simulink model "sm_DynamicCompression"  (R2019b)
settings: Solver=FixedStepDiscrete  StartTime=0.0  StopTime=stop_time  RelTol=1e-3
InitFcn:
  | sm_callback_init
StopFcn:
  | sm_callback_stop
values from neighbouring files (symbols this model uses):
  a = 100*(r^2)    [InitializeCompressionSettings.m]    (also in sm_check_control_signals.m = registers(i).(supplied_fields{j}); sm_check_control_signals_LOCAL_1434.m = registers(i).(supplied_fields{j}))
  B_k_0_init = zeros(1,FIR_0_Uprate)    [sm_callback_init.m]
  B_k_1_init = zeros(1,FIR_0_Uprate)    [sm_callback_init.m]
  B_k_2_init = zeros(1,FIR_0_Uprate)    [sm_callback_init.m]
  B_k_3_init = zeros(1,FIR_0_Uprate)    [sm_callback_init.m]
  B_k_4_init = zeros(1,FIR_0_Uprate)    [sm_callback_init.m]
  B_k_5_init = zeros(1,FIR_0_Uprate)    [sm_callback_init.m]
  calib_bpfs = bpfs    [sm_compression_init.m]
  delayFix = maxDelay-delays    [Initialize_Delay_Values.m]
  F_bits = 28    [TestingLibraryScripts.m]    (also in sm_compression_init.m)
  FIR_0_Size = (ceil(log2(length(calib_bpfs(2:calib_bpfs(1,1)+1 ,1)'))))    [sm_callback_init.m]
  FIR_0_Uprate = 2^FIR_0_Size    [sm_callback_init.m]
  M_bits = 1    [TestingLibraryScripts.m]    (also in sm_compression_init.m = 5)
  M_Bits = M_bits    (= 5)    [sm_compression_init.m]
  mp = sm_init_avalon_signals(mp)    [sm_callback_init.m]
  r_att = nthroot(0.1, s_att)    [sm_compression_init.m]
  r_rel = nthroot(0.1, s_rel)    [sm_compression_init.m]
  recombGain = ones(1,NChans)    [sm_compression_init.m]
  TABLE_SEL_BYPASS_ENABLE = 0    [sm_callback_init.m]
  Ts = mp.Ts    [sm_compression_init.m]
  Ts_system = mp.Ts_system    [sm_compression_init.m]
  W_bits = 32    [TestingLibraryScripts.m]    (also in sm_compression_init.m)
  X_high = 1    [sm_compression_init.m]
undefined symbols (not defined in the file or in its folder): b, c, Gain_Table, ig_eq
libraries: hdlsllib x272, simulink x127, dsphdlfiltering x2
(part 1 of 8)
settings Model: Creator=Ross  LastModifiedBy=cb54103
settings DataIOCC: ReturnWorkspaceOutputs=off
settings OptimizationCC: BlockReduction=off  ConditionallyExecuteInputs=off  DefaultParameterBehavior=Inlined
settings DebuggingCC: ReadBeforeWriteMsg=DisableAll  WriteAfterWriteMsg=DisableAll  WriteAfterReadMsg=DisableAll  AlgebraicLoopMsg=error  MultiTaskDSMMsg=none  SingleTaskRateTransMsg=error  PregeneratedLibrarySubsystemCodeDiagnostic=none  ArithmeticOperatorsInVariantConditions=warning
settings HardwareCC: ProdBitPerPointer=32  ProdBitPerSizeT=32  ProdBitPerPtrDiffT=32  ProdLargestAtomicFloat=None  ProdIntDivRoundTo=Undefined  ProdEndianess=Unspecified  ProdWordSize=32  ProdHWDeviceType=ASIC/FPGA->ASIC/FPGA  TargetBitPerLong=64  TargetBitPerPointer=64  TargetBitPerSizeT=64  TargetBitPerPtrDiffT=64  TargetLongLongMode=on  TargetIntDivRoundTo=Zero  TargetEndianess=LittleEndian  TargetWordSize=64  TargetHWDeviceType=Custom Processor->MATLAB Host Computer  ProdEqTarget=off
settings ModelReferenceCC: UpdateModelReferenceTargets=IfOutOfDate
settings SFSimCC: SFSimEcho=off  SimUseLocalCustomCode=off  CustomCodeUndefinedFunction=UseInterfaceOnly
settings RTWCC: RTWUseLocalCustomCode=off

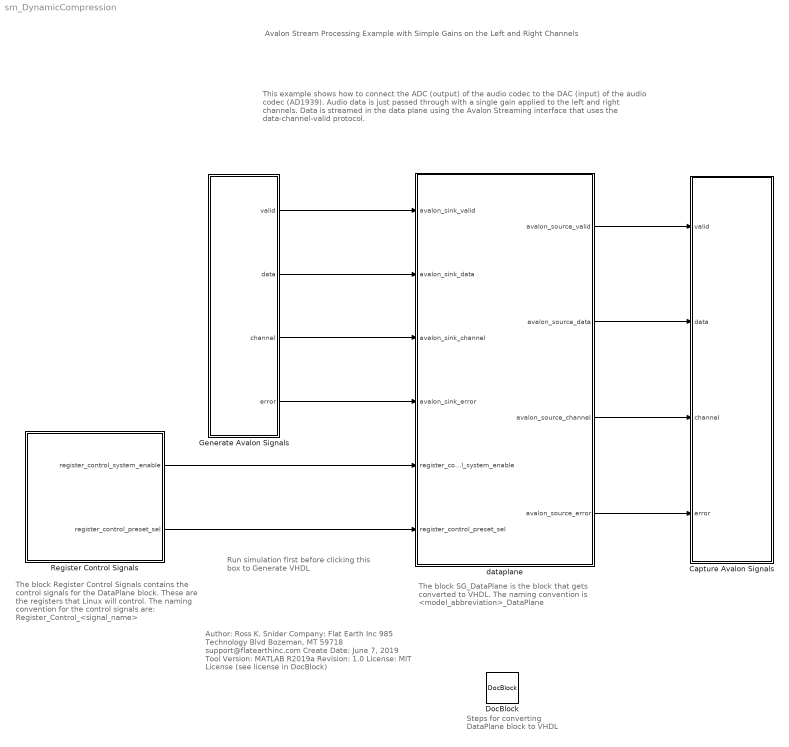
== system sm_DynamicCompression ==
  note: The block SG_DataPlane is the block that gets
      | converted to VHDL. The naming convention is
      | <model_abbreviation>_DataPlane
  note: Author:          Ross K. Snider
      | Company:     Flat Earth Inc
      |                       985 Technology Blvd
      |                       Bozeman, MT 59718
      |                       support@flatearthinc.com
      | Create Date:  June 7, 2019
      | Tool Version:  MATLAB R2019a
      | Revision:        1.0
      | License:          MIT License (see license in DocBlock)
  note: This example shows how to connect the ADC (output) of the audio codec to the DAC (input) of the audio codec (AD1939). Audio data is just passed through with a single gain applied to the left and right channels. Data is streamed in the data plane using the Avalon Streaming interface that uses the data-channel-valid protocol.
  note: Steps for converting
      | DataPlane block
      | to VHDL
  note: Avalon Stream Processing Example
      | with Simple Gains on the Left and Right Channels
  note: Run simulation first
      | before clicking this box to
      | Generate VHDL
  note: The block Register Control Signals contains
      | the control signals for the DataPlane block.
      | These are the registers that Linux will control.
      | The naming convention for the control
      | signals are:  Register_Control_<signal_name>
  Capture Avalon Signals : Subsystem
  DocBlock : simulink/Model-Wide Utilities/DocBlock  DocumentType=HTML
      content=|
      | <html><head></head><body>
      | Type your documentation here</body></html>
  Generate Avalon Signals : Subsystem
  Register Control Signals : Subsystem
  dataplane : Subsystem  TreatAsAtomicUnit=on
  wires:
  Generate Avalon Signals/2(data) -> dataplane/2(avalon_sink_data)
  Generate Avalon Signals/1(valid) -> dataplane/1(avalon_sink_valid)
  Generate Avalon Signals/3(channel) -> dataplane/3(avalon_sink_channel)
  Generate Avalon Signals/4(error) -> dataplane/4(avalon_sink_error)
  dataplane/2(avalon_source_data) -> Capture Avalon Signals/2(data)
  dataplane/1(avalon_source_valid) -> Capture Avalon Signals/1(valid)
  dataplane/3(avalon_source_channel) -> Capture Avalon Signals/3(channel)
  dataplane/4(avalon_source_error) -> Capture Avalon Signals/4(error)
  Register Control Signals/1(register_control_system_enable) -> dataplane/5(register_control_system_enable)
  Register Control Signals/2(register_control_preset_sel) -> dataplane/6(register_control_preset_sel)

== system sm_DynamicCompression/Capture Avalon Signals ==
  note: Note:  If these "To Workspace" variables show up under a variable called "out",
      | Open the Configure Logging... window (Simulation->Output->Configure Logging...)
      | and deselect the checkbox "Single simulation output:" found under the "Save to workspace or file" section.
  valid : Inport
  data : Inport  Port=2
  channel : Inport  Port=3
  error : Inport  Port=4
  To Workspace : ToWorkspace  VariableName=Avalon_Sink_Data  SaveFormat=Timeseries  SampleTime=-1
  To Workspace1 : ToWorkspace  VariableName=Avalon_Sink_Valid  SaveFormat=Timeseries  SampleTime=-1
  To Workspace2 : ToWorkspace  VariableName=Avalon_Sink_Channel  SaveFormat=Timeseries  SampleTime=-1
  To Workspace3 : ToWorkspace  VariableName=Avalon_Sink_Error  SaveFormat=Timeseries  SampleTime=-1
  wires:
  data/1 -> To Workspace/1
  valid/1 -> To Workspace1/1
  error/1 -> To Workspace3/1
  channel/1 -> To Workspace2/1

== system sm_DynamicCompression/Generate Avalon Signals ==
  note: Avalon Streaming Sink Signals
      | Note: We are assuming a specific system clock frequency that these signals are being clock in at.
      | The interface needs to be regenerated if this system clock frequency changes. Change system clock frequency in InitFcn callback in Model Explorer.
      |
      | -- Avalon streaming slave interface (sink)
      | AD1939_DAC_data : in std_logic_vector(31 downto 0); -- W=32; F=28; Signed 2's Complement
      | AD1939_DAC_channel : in std_logic_vector(1 downto 0); -- Left <-> channel 0; Right <-> channel 1 (other two channels are ignored)
      | AD1939_DAC_valid : in std_logic; -- asserted when data is valid
      | AD1939_DAC_error : in std_logic_vector(1 downto 0) -- error channel is ignored, assumed to be error free at this point
      |
      | For more information on the data-channel-valid protocol, see chapter 5 in Intel's Avalon Interfaced Specification (p. 40) at https://www.intel.com/content/dam/www/programmable/us/en/pdfs/literature/manual/mnl_avalon_spec.pdf
  Avalon Source Channel : FromWorkspace  VariableName=mp.Avalon_Source_Channel  OutDataTypeStr=double  SampleTime=mp.Ts_system
  "Avalon Source Data " : FromWorkspace  VariableName=mp.Avalon_Source_Data  OutDataTypeStr=double  SampleTime=mp.Ts_system
  Avalon Source Error : FromWorkspace  VariableName=mp.Avalon_Source_Error  OutDataTypeStr=double  SampleTime=mp.Ts_system
  Avalon Source Valid : FromWorkspace  VariableName=mp.Avalon_Source_Valid  OutDataTypeStr=double  SampleTime=mp.Ts_system
  Data Type Conversion : DataTypeConversion  OutDataTypeStr=fixdt(1,mp.W_bits,mp.F_bits)
  Data Type Conversion1 : DataTypeConversion  OutDataTypeStr=fixdt(0,2,0)
  Data Type Conversion2 : DataTypeConversion  OutDataTypeStr=boolean
  Data Type Conversion3 : DataTypeConversion  OutDataTypeStr=fixdt(0,2,0)
  valid : Outport  VectorParamsAs1DForOutWhenUnconnected=off
  data : Outport  Port=2  VectorParamsAs1DForOutWhenUnconnected=off
  channel : Outport  Port=3  VectorParamsAs1DForOutWhenUnconnected=off
  error : Outport  Port=4  VectorParamsAs1DForOutWhenUnconnected=off
  wires:
  Data Type Conversion1/1 -> channel/1
  Data Type Conversion2/1 -> valid/1
  Avalon Source Error/1 -> Data Type Conversion3/1
  Data Type Conversion/1 -> data/1
  Avalon Source Valid/1 -> Data Type Conversion2/1
  Data Type Conversion3/1 -> error/1
  Avalon Source Channel/1 -> Data Type Conversion1/1
  "Avalon Source Data "/1 -> Data Type Conversion/1

== system sm_DynamicCompression/Register Control Signals ==
  note: Control Signals that will be coming from Linux via
      | memory mapped registers need to have names
      | containing the prefix "register_control_"
      | (all lower case)
  Data Type Conversion1 : DataTypeConversion  OutDataTypeStr=fixdt(1,mp.W_bits,mp.F_bits)
  Data Type Conversion2 : DataTypeConversion  OutDataTypeStr=fixdt(1,mp.W_bits,mp.F_bits)
  Time Series Signal from Workspace 1 : FromWorkspace  VariableName=mp.register(1).timeseries  OutDataTypeStr=double  SampleTime=mp.Ts_system
  Time Series Signal from Workspace 2 : FromWorkspace  VariableName=mp.register(2).timeseries  OutDataTypeStr=double  SampleTime=mp.Ts_system
  register_control_system_enable : Outport  VectorParamsAs1DForOutWhenUnconnected=off
  register_control_preset_sel : Outport  Port=2  VectorParamsAs1DForOutWhenUnconnected=off
  wires:
  Time Series Signal from Workspace 1/1 -> Data Type Conversion2/1
  Time Series Signal from Workspace 2/1 -> Data Type Conversion1/1
  Data Type Conversion2/1 -> register_control_system_enable/1
  Data Type Conversion1/1 -> register_control_preset_sel/1

== system sm_DynamicCompression/dataplane ==
  note: Control Signals that will be coming from Linux via
      | memory mapped registers need to have names
      | containing the prefix "register_control_"
      | (all lower case)
  note: The Avalon Data Processing Block
      | performs DSP on the left and right channels.
  note: The Avalon Data Processing block
      | only executes when valid is asserted
  note: Ignore Errors.
      | Assuming no errors coming from the ADC and errors going to DAC will be ignored.
      | Any Error streaming needs to be done inside Avalon Data Processing block.
  note: Avalon streaming interface signals need to have the
      | names containing the prefix "avalon_"
      | (all lower case)
  avalon_sink_valid : Inport
  avalon_sink_data : Inport  Port=2
  avalon_sink_channel : Inport  Port=3
  avalon_sink_error : Inport  Port=4
  register_control_system_enable : Inport  Port=5
  register_control_preset_sel : Inport  Port=6
  Avalon Data Processing : Subsystem  TreatAsAtomicUnit=on
  avalon_source_valid : Outport  VectorParamsAs1DForOutWhenUnconnected=off
  avalon_source_data : Outport  Port=2  VectorParamsAs1DForOutWhenUnconnected=off
  avalon_source_channel : Outport  Port=3  VectorParamsAs1DForOutWhenUnconnected=off
  avalon_source_error : Outport  Port=4  VectorParamsAs1DForOutWhenUnconnected=off
  wires:
  avalon_sink_channel/1 -> Avalon Data Processing/3(Sink_Channel)
  avalon_sink_error/1 -> avalon_source_error/1
  Avalon Data Processing/1(Source_Data) -> avalon_source_data/1
  avalon_sink_valid/1 -> avalon_source_valid/1, Avalon Data Processing/1(Sink_Valid)
  avalon_sink_data/1 -> Avalon Data Processing/2(Sink_Data)
  Avalon Data Processing/2(Source_Channel) -> avalon_source_channel/1
  register_control_preset_sel/1 -> Avalon Data Processing/5(Register_Preset_Sel)
  register_control_system_enable/1 -> Avalon Data Processing/4(Register_System_Enable)

== system sm_DynamicCompression/dataplane/Avalon Data Processing ==
  note: Select output data
      | based on channel number
  note: Check if Channel 0
      | (Left Channel)
  note: The Left Channel Processing block
      | only executes when channel 0
      | is detected
  note: The Right Channel Processing block
      | only executes when channel 1
      | is detected
  note: Check if Channel 1
      | (Right Channel)
  Sink_Valid : Inport
  Sink_Data : Inport  Port=2
  Sink_Channel : Inport  Port=3
  Register_System_Enable : Inport  Port=4
  Register_Preset_Sel : Inport  Port=5
  Compare To Constant1 : simulink/Logic and Bit Operations/Compare To Constant  relop===  const=1  OutDataTypeStr=boolean
  Compare To Constant2 : simulink/Logic and Bit Operations/Compare To Constant  relop===  const=0  OutDataTypeStr=boolean
  Left Channel Processing : Subsystem  TreatAsAtomicUnit=on
  Logical Operator : Logic  AllPortsSameDT=off  OutDataTypeStr=boolean
  Multiport Switch : MultiPortSwitch  DataPortOrder=Zero-based contiguous  DiagnosticForDefault=None  zeroidx=on
  Right Channel Processing : Subsystem  TreatAsAtomicUnit=on
  Source_Data : Outport  InitialOutput=0  VectorParamsAs1DForOutWhenUnconnected=off
  Source_Channel : Outport  Port=2  InitialOutput=0  VectorParamsAs1DForOutWhenUnconnected=off
  wires:
  Sink_Channel/1 -> Source_Channel/1, Multiport Switch/1, Compare To Constant1/1, Compare To Constant2/1
  Compare To Constant1/1 -> Right Channel Processing/Enable
  Sink_Data/1 -> Multiport Switch/4, Right Channel Processing/1(Right_Data_In), Left Channel Processing/1(Left_Data_In)
  Left Channel Processing/1("Left_Data_Out ") -> Multiport Switch/2
  Right Channel Processing/1("Right_Data_Out ") -> Multiport Switch/3
  Multiport Switch/1 -> Source_Data/1
  Register_System_Enable/1 -> Left Channel Processing/2(Register_System_Enable)
  Register_Preset_Sel/1 -> Left Channel Processing/3(Register_Preset_Sel), Right Channel Processing/2(Right_Gain)
  Logical Operator/1 -> Left Channel Processing/4(Valid_in)
  Compare To Constant2/1 -> Logical Operator/2
  Sink_Valid/1 -> Logical Operator/1

== system sm_DynamicCompression/dataplane/Avalon Data Processing/Left Channel Processing ==
  note: Put in a check here if we make L/R channels have different tables
  Left_Data_In : Inport
  Register_System_Enable : Inport  Port=2
  Register_Preset_Sel : Inport  Port=3
  Valid_in : Inport  Port=4
  Cast To Boolean : DataTypeConversion  Commented=on  OutDataTypeStr=boolean
  Cast To Boolean1 : DataTypeConversion  Commented=on  OutDataTypeStr=boolean
  Cast To fp(1,32,28) : DataTypeConversion  Commented=on  OutDataTypeStr=fixdt(1,32,28)  RndMeth=Round
  Cast To fp(1,32,28)1 : DataTypeConversion  Commented=on  OutDataTypeStr=fixdt(1,32,28)  RndMeth=Round
  Constant2 : Constant  Value=0  OutDataTypeStr=boolean  SampleTime=-1
  From Workspace : FromWorkspace  Commented=on  VariableName=sig_in  SampleTime=Ts  OutputAfterFinalValue=Setting to zero
  From Workspace1 : FromWorkspace  Commented=on  VariableName=Table_Fill_t  SampleTime=Ts  Interpolate=off  OutputAfterFinalValue=Setting to zero
  From Workspace2 : FromWorkspace  Commented=on  VariableName=Fill_Valid_t  SampleTime=Ts  OutputAfterFinalValue=Setting to zero
  From Workspace4 : FromWorkspace  Commented=on  VariableName=Reset  SampleTime=Ts  Interpolate=off  OutputAfterFinalValue=Setting to zero
  Switch : Switch
  Terminator{,1..3} (4 alike) : Terminator  Commented=on
  To Workspace : ToWorkspace  Commented=on  VariableName=proc_sig  SaveFormat=Timeseries  SampleTime=-1
  recalculate : Subsystem
  "Left_Data_Out " : Outport  InitialOutput=0  VectorParamsAs1DForOutWhenUnconnected=off
  wires:
  Cast To Boolean1/1 -> Terminator3/1
  Cast To Boolean/1 -> Terminator2/1
  Cast To fp(1,32,28)1/1 -> Terminator/1
  From Workspace1/1 -> Cast To fp(1,32,28)/1  "Table_Values"
  recalculate/1(proc_sig) -> Switch/1, To Workspace/1
  From Workspace2/1 -> Cast To Boolean/1
  From Workspace/1 -> Cast To fp(1,32,28)1/1
  From Workspace4/1 -> Cast To Boolean1/1
  Cast To fp(1,32,28)/1 -> Terminator1/1
  Left_Data_In/1 -> Switch/3, recalculate/4(sig)
  Constant2/1 -> recalculate/6(Memory_Reset)
  Register_System_Enable/1 -> recalculate/1(Register_Data), Switch/2
  Register_Preset_Sel/1 -> recalculate/2(Register_Addr), recalculate/3(Register_Preset_Sel)
  Valid_in/1 -> recalculate/5(Valid_in)
  Switch/1 -> "Left_Data_Out "/1

== system sm_DynamicCompression/dataplane/Avalon Data Processing/Right Channel Processing ==
  note: Apply Right Gain
  note: An enabled subsystem
      | This subsystem only runs when the data valid signal is enabled (asserted)
  Right_Data_In : Inport
  Right_Gain : Inport  Port=2
  Enable : EnablePort
  Data Type Conversion : DataTypeConversion  OutDataTypeStr=fixdt(1,mp.W_bits,mp.F_bits)
  Product : Product
  "Right_Data_Out " : Outport  InitialOutput=0  VectorParamsAs1DForOutWhenUnconnected=off
  wires:
  Data Type Conversion/1 -> "Right_Data_Out "/1
  Product/1 -> Data Type Conversion/1
  Right_Data_In/1 -> Product/1
  Right_Gain/1 -> Product/2

== system sm_DynamicCompression/dataplane/Avalon Data Processing/Left Channel Processing/recalculate ==
  note: High Clipping
  note: Prescription Application
  note: Low Clipping
  Register_Data : Inport
  Register_Addr : Inport  Port=2
  Register_Preset_Sel : Inport  Port=3
  sig : Inport  Port=4
  Valid_in : Inport  Port=5
  Memory_Reset : Inport  Port=6
  Compare To Constant : simulink/Logic and Bit Operations/Compare To Constant  relop=>=  const=X_high  OutDataTypeStr=boolean
  Compare To Constant1 : simulink/Logic and Bit Operations/Compare To Constant  relop=<=  const=-X_high  OutDataTypeStr=boolean
  Constant : Constant  Value=X_high  OutDataTypeStr=fixdt(1,W_bits, F_bits)  SampleTime=-1
  Constant1 : Constant  Value=-X_high  OutDataTypeStr=fixdt(1,W_bits, F_bits)  SampleTime=-1
  Nchan_FbankAGC_AID : Subsystem
  Static_pFIR : Subsystem
  Switch : Switch  Criteria=u2 ~= 0
  Switch1 : Switch  Criteria=u2 ~= 0
  ig65 fir : DiscreteFir  Commented=on  Coefficients=ig_eq  CoefDataTypeStr=fixdt(1, W_bits*2, W_bits)  ProductDataTypeStr=fixdt(1, W_bits*2, W_bits)  AccumDataTypeStr=fixdt(1, W_bits*2, W_bits)  OutDataTypeStr=fixdt(1, W_bits, F_bits)
  proc_sig : Outport  VectorParamsAs1DForOutWhenUnconnected=off
  wires:
  sig/1 -> Nchan_FbankAGC_AID/4(input_signal)
  Register_Data/1 -> Nchan_FbankAGC_AID/1(Register_Data)
  Register_Addr/1 -> Nchan_FbankAGC_AID/2(Register_Addr)
  Memory_Reset/1 -> Nchan_FbankAGC_AID/6(Reset)
  Static_pFIR/1(Data_out) -> Compare To Constant/1, Switch/3  "re_level.*eq_sig"
  Nchan_FbankAGC_AID/1(proc_sig) -> Static_pFIR/1(Compressed_Data_In)
  Compare To Constant/1 -> Switch/2
  Constant/1 -> Switch/1
  Switch/1 -> Switch1/3, Compare To Constant1/1
  Compare To Constant1/1 -> Switch1/2
  Constant1/1 -> Switch1/1
  Switch1/1 -> proc_sig/1
  Valid_in/1 -> Nchan_FbankAGC_AID/5(Valid_in)
  Nchan_FbankAGC_AID/2(Valid_out) -> Static_pFIR/2(Valid_in)
  Register_Preset_Sel/1 -> Nchan_FbankAGC_AID/3(Register_Preset_Sel)

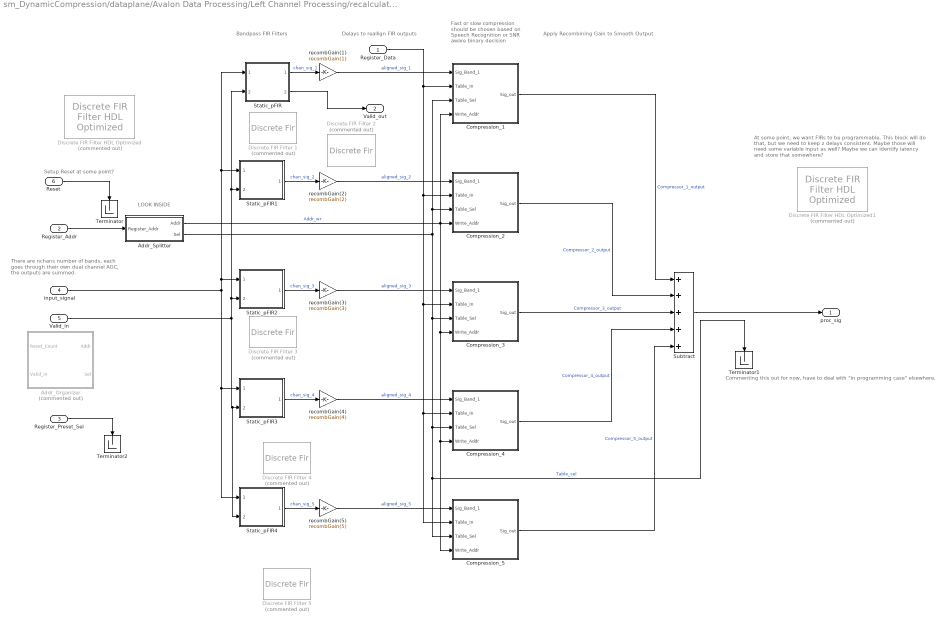
== system sm_DynamicCompression/dataplane/Avalon Data Processing/Left Channel Processing/recalculate/Nchan_FbankAGC_AID ==
  note: LOOK INSIDE
  note: Commenting this out for now, have to deal with "in programming case" elsewhere.
  note: At some point, we want FIRs to be programmable.
      | This block will do that, but we need to keep z delays consistent.
      | Maybe those will need some variable input as well?
      | Maybe we can identify latency and store that somewhere?
  note: Setup Reset at some point?
  note: Apply Recombining Gain to Smooth Output
  note: Fast or slow compression
      | should be chosen based
      | on Speech Recognition or
      | SNR aware binary decision
  note: Delays to reallign FIR outputs
  note: Bandpass FIR Filters
  note: There are nchans number of bands,
      |  each goes through their own dual
      | channel AGC, the outputs are summed.
  Register_Data : Inport
  Register_Addr : Inport  Port=2
  Register_Preset_Sel : Inport  Port=3
  input_signal : Inport  Port=4
  Valid_in : Inport  Port=5
  Reset : Inport  Port=6
  Addr_Organizer : Subsystem  Commented=on
  Addr_Splitter : Subsystem
  Compression_1 : Subsystem
  Compression_2 : Subsystem
  Compression_3 : Subsystem
  Compression_4 : Subsystem
  Compression_5 : Subsystem
  Discrete FIR Filter HDL Optimized : dsphdlfiltering/Discrete FIR Filter HDL Optimized  Commented=on  NumeratorSource=Property  Numerator=[ 0.5, 0.5 ]  NumeratorPrototype=[ 0.5, 0.5 ]  FilterStructure=Direct form systolic  SerializationOption=Minimum number of cycles between valid input samples  NumberOfCycles=2  NumberOfMultipliers=2  SimulateUsing=Code generation  roundingMode=Floor  overflowMode=off  CoefficientsDataTypeStr=Inherit: Same word length as input  CoefficientsMin=[]  CoefficientsMax=[]  OutputMin=[]  OutputMax=[]  ResetInputPort=off  HDLGlobalReset=off
      settings: SourceProductName=DSP System Toolbox  SourceProductBaseCode=DS
  Discrete FIR Filter HDL Optimized1 : dsphdlfiltering/Discrete FIR Filter HDL Optimized  Commented=on  NumeratorSource=Input port (Parallel interface)  Numerator=[ 0.5, 0.5 ]  NumeratorPrototype=[ 0.5, 0.5 ]  FilterStructure=Direct form systolic  SerializationOption=Minimum number of cycles between valid input samples  NumberOfCycles=2  NumberOfMultipliers=2  SimulateUsing=Code generation  roundingMode=Floor  overflowMode=off  CoefficientsDataTypeStr=Inherit: Same word length as input  CoefficientsMin=[]  CoefficientsMax=[]  OutputMin=[]  OutputMax=[]  ResetInputPort=off  HDLGlobalReset=off
      settings: SourceProductName=DSP System Toolbox  SourceProductBaseCode=DS
  Discrete FIR Filter 1 : DiscreteFir  Commented=on  Coefficients=calib_bpfs(2:calib_bpfs(1,1)+1 ,1)'  CoefDataTypeStr=fixdt(1, W_bits, F_bits)  ProductDataTypeStr=fixdt(1, W_bits, F_bits)  AccumDataTypeStr=fixdt(1, W_bits, F_bits)  OutDataTypeStr=fixdt(1, W_bits, F_bits)
  Discrete FIR Filter 2 : DiscreteFir  Commented=on  Coefficients=calib_bpfs(2:calib_bpfs(1,2)+1 ,2)'  CoefDataTypeStr=fixdt(1, W_bits, F_bits)  ProductDataTypeStr=fixdt(1, W_bits, F_bits)  AccumDataTypeStr=fixdt(1, W_bits, F_bits)  OutDataTypeStr=fixdt(1, W_bits, F_bits)
  Discrete FIR Filter 3 : DiscreteFir  Commented=on  Coefficients=calib_bpfs(2:calib_bpfs(1,3)+1 ,3)'  CoefDataTypeStr=fixdt(1, W_bits, F_bits)  ProductDataTypeStr=fixdt(1, W_bits, F_bits)  AccumDataTypeStr=fixdt(1, W_bits, F_bits)  OutDataTypeStr=fixdt(1, W_bits, F_bits)
  Discrete FIR Filter 4 : DiscreteFir  Commented=on  Coefficients=calib_bpfs(2:calib_bpfs(1,4)+1 ,4)'  CoefDataTypeStr=fixdt(1, W_bits, F_bits)  ProductDataTypeStr=fixdt(1, W_bits, F_bits)  AccumDataTypeStr=fixdt(1, W_bits, F_bits)  OutDataTypeStr=fixdt(1, W_bits, F_bits)
  Discrete FIR Filter 5 : DiscreteFir  Commented=on  Coefficients=calib_bpfs(2:calib_bpfs(1,5)+1 ,5)'  CoefDataTypeStr=fixdt(1, W_bits, F_bits)  ProductDataTypeStr=fixdt(1, W_bits, F_bits)  AccumDataTypeStr=fixdt(1, W_bits, F_bits)  OutDataTypeStr=fixdt(1, W_bits, F_bits)
  Static_pFIR : Subsystem
  Static_pFIR1 : Subsystem
  Static_pFIR2 : Subsystem
  Static_pFIR3 : Subsystem
  Static_pFIR4 : Subsystem
  Subtract : Sum  Inputs=+++++
  Terminator : Terminator
  Terminator1 : Terminator
  Terminator2 : Terminator
  recombGain(1) : Gain  Gain=recombGain(1)  OutDataTypeStr=Inherit: Same as input
  recombGain(2) : Gain  Gain=recombGain(2)  OutDataTypeStr=Inherit: Same as input
  recombGain(3) : Gain  Gain=recombGain(3)  OutDataTypeStr=Inherit: Same as input
  recombGain(4) : Gain  Gain=recombGain(4)  OutDataTypeStr=Inherit: Same as input
  recombGain(5) : Gain  Gain=recombGain(5)  OutDataTypeStr=Inherit: Same as input
  proc_sig : Outport  VectorParamsAs1DForOutWhenUnconnected=off
  Valid_out : Outport  Port=2  VectorParamsAs1DForOutWhenUnconnected=off
  wires:
  Static_pFIR/1(Data_out) -> recombGain(1)/1  "chan_sig_1"
  recombGain(1)/1 -> Compression_1/1(Sig_Band_1)  "aligned_sig_1"
  Compression_1/1(Sig_out) -> Subtract/1  "Compressor_1_output"
  recombGain(2)/1 -> Compression_2/1(Sig_Band_1)  "aligned_sig_2"
  Static_pFIR1/1(Data_out) -> recombGain(2)/1  "chan_sig_2"
  recombGain(3)/1 -> Compression_3/1(Sig_Band_1)  "aligned_sig_3"
  Static_pFIR2/1(Data_out) -> recombGain(3)/1  "chan_sig_3"
  Static_pFIR4/1(Data_out) -> recombGain(5)/1  "chan_sig_5"
  input_signal/1 -> Static_pFIR2/1(Data_In), Static_pFIR1/1(Data_In), Static_pFIR/1(Data_In), Static_pFIR4/1(Data_In), Static_pFIR3/1(Data_In)
  recombGain(5)/1 -> Compression_5/1(Sig_Band_1)  "aligned_sig_5"
  recombGain(4)/1 -> Compression_4/1(Sig_Band_1)  "aligned_sig_4"
  Static_pFIR3/1(Data_out) -> recombGain(4)/1  "chan_sig_4"
  Compression_3/1(Sig_out) -> Subtract/3  "Compressor_3_output"
  Compression_2/1(Sig_out) -> Subtract/2  "Compressor_2_output"
  Compression_4/1(Sig_out) -> Subtract/4  "Compressor_4_output"
  Compression_5/1(Sig_out) -> Subtract/5  "Compressor_5_output"
  Addr_Splitter/1(Addr) -> Compression_3/4(Write_Addr), Compression_5/4(Write_Addr), Compression_4/4(Write_Addr), Compression_2/4(Write_Addr), Compression_1/4(Write_Addr)  "Addr_wr"
  Reset/1 -> Terminator/1
  Register_Addr/1 -> Addr_Splitter/1(Register_Addr)
  Register_Data/1 -> Compression_5/2(Table_In), Compression_4/2(Table_In), Compression_3/2(Table_In), Compression_2/2(Table_In), Compression_1/2(Table_In)
  Addr_Splitter/2(Sel) -> Compression_3/3(Table_Sel), Terminator1/1, Compression_5/3(Table_Sel), Compression_4/3(Table_Sel), Compression_1/3(Table_Sel), Compression_2/3(Table_Sel)  "Table_sel"
  Subtract/1 -> proc_sig/1
  Valid_in/1 -> Static_pFIR4/2(Valid_in), Static_pFIR3/2(Valid_in), Static_pFIR2/2(Valid_in), Static_pFIR/2(Valid_in), Static_pFIR1/2(Valid_in)
  Static_pFIR/2(Valid_out) -> Valid_out/1
  Register_Preset_Sel/1 -> Terminator2/1

== system sm_DynamicCompression/dataplane/Avalon Data Processing/Left Channel Processing/recalculate/Static_pFIR ==
  note: consider desired output rate
  note: B_ks will be programmable eventually.
      | For the Conference, they will be preset.
  Compressed_Data_In : Inport
  Valid_in : Inport  Port=2
  "Addr_Gen " : Subsystem
  Alignment_Delay : UnitDelay  SampleTime=-1  HasFrameUpgradeWarning=on
  Always_read_B2 : Constant  Value=0  OutDataTypeStr=boolean  SampleTime=Ts/FIR_0_Uprate
  B_k_Memory_Block2 : Subsystem  AncestorBlock=DualPortRam_UNLOCKED/Dual Rate Dual Port RAM1  mask(Dual-rate dual-port RAM){ram_size=FIR_0_Size}
      mask prompts: ram_size "Address port width (2 to 28 bits)"
      mask help: This block simulates a dual-clock dual-port RAM with two data output ports.
      mask init:
      | hdlblkmask_drdpram();
      mask Help: helpview([docroot '/simulink/helptargets.map'],'HDL_dual_rate_dual_port_ram');
  Input_Data_Circular_Buffer : hdlsllib/HDL RAMs/Simple Dual Port RAM  ram_size=FIR_0_Size
      settings: SourceProductName=Simulink  SourceProductBaseCode=SL
  Input_Data_Circular_Buffer_old : Subsystem  Commented=on  AncestorBlock=DualPortRam_UNLOCKED/Dual Rate Dual Port RAM1  mask(Dual-rate dual-port RAM){ram_size=FIR_0_Size}
      mask prompts: ram_size "Address port width (2 to 28 bits)"
      mask help: This block simulates a dual-clock dual-port RAM with two data output ports.
      mask init:
      | hdlblkmask_drdpram();
      mask Help: helpview([docroot '/simulink/helptargets.map'],'HDL_dual_rate_dual_port_ram');
  Multiply_And_Sum : Subsystem
  Never_write_B2 : Constant  Value=0  OutDataTypeStr=fixdt(1, W_bits*2, W_bits)  SampleTime=Ts/FIR_0_Uprate
  Output_memory : UnitDelay  SampleTime=-1  HasFrameUpgradeWarning=on
  READ_ONLY_1 : Constant  Value=0  OutDataTypeStr=fixdt(1, W_bits*2, W_bits)  SampleTime=Ts/FIR_0_Uprate
  READ_ONLY_2 : Constant  Value=0  OutDataTypeStr=fixdt(0,FIR_0_Size, 0)  SampleTime=Ts/FIR_0_Uprate
  READ_ONLY_3 : Constant  Value=0  OutDataTypeStr=boolean  SampleTime=Ts/FIR_0_Uprate
  Rate Transition : RateTransition  Commented=on  OutPortSampleTime=Ts
  Reset_Switch : Switch  Criteria=u2 ~= 0
  Terminator7 : Terminator
  Data_out : Outport  VectorParamsAs1DForOutWhenUnconnected=off
  wires:
  READ_ONLY_2/1 -> B_k_Memory_Block2/2(addr_A)
  Always_read_B2/1 -> B_k_Memory_Block2/6(we_B)
  B_k_Memory_Block2/1(dout_A) -> Terminator7/1
  "Addr_Gen "/3(End_of_sample_calc) -> Alignment_Delay/1
  B_k_Memory_Block2/2(dout_B) -> Multiply_And_Sum/3(b_i)  "b_i"
  Reset_Switch/1 -> Output_memory/1
  Multiply_And_Sum/2(Output_Valid) -> Reset_Switch/2
  READ_ONLY_1/1 -> B_k_Memory_Block2/1(din_A)
  Never_write_B2/1 -> B_k_Memory_Block2/4(din_B)
  Input_Data_Circular_Buffer/1 -> Multiply_And_Sum/1(x[n-i])  "x[n-i]"
  "Addr_Gen "/2(Data_History_Rd_addr) -> Input_Data_Circular_Buffer/4
  Valid_in/1 -> Input_Data_Circular_Buffer/3
  Output_memory/1 -> Data_out/1, Reset_Switch/3
  READ_ONLY_3/1 -> B_k_Memory_Block2/3(we_A)
  "Addr_Gen "/1(Input_Addr) -> Input_Data_Circular_Buffer/2
  Multiply_And_Sum/1(Filtered_Output) -> Reset_Switch/1
  "Addr_Gen "/4(b_k_addr) -> B_k_Memory_Block2/5(addr_B)
  Compressed_Data_In/1 -> Input_Data_Circular_Buffer/1  "x[n]"
  Alignment_Delay/1 -> Multiply_And_Sum/2(End_of_sample_calc)

== system sm_DynamicCompression/dataplane/Avalon Data Processing/Left Channel Processing/recalculate/Nchan_FbankAGC_AID/Addr_Organizer ==
  note: Addr line contains the local address bits: 0-63
  note: Select Line is 000 to 101, if 110 writing is complete
  Reset_Count : Inport
  Valid_in : Inport  Port=2
  Bit Slice : hdlsllib/Logic and Bit Operations/Bit Slice  lidx=3+M_bits  ridx=0
      settings: SourceProductName=Simulink  SourceProductBaseCode=SL
  Bit Slice1 : hdlsllib/Logic and Bit Operations/Bit Slice  lidx=6+M_bits  ridx=4+M_bits
      settings: SourceProductName=Simulink  SourceProductBaseCode=SL
  Counter_up_to_320 : hdlsllib/Sources/HDL Counter  CountType=Count limited  CountInit=5*2^(4+M_Bits)  CountStep=1  CountMax=5*2^(4+M_Bits)+1  CountFromType=Initial value  CountFrom=5*2^(4+M_Bits)  CountResetPort=on  CountLoadPort=off  CountEnbPort=on  CountDirPort=off  CountDataType=Unsigned  CountWordLen=7+M_Bits  CountFracLen=0  CountSampTime=1
      settings: SourceProductName=Simulink
  Data Type Conversion : DataTypeConversion  OutDataTypeStr=fixdt(0,7+M_Bits,0)
  Data Type Conversion1 : DataTypeConversion  OutDataTypeStr=fixdt(0,4+M_bits,0)
  Data Type Conversion2 : DataTypeConversion  OutDataTypeStr=fixdt(0,3,0)
  Addr : Outport  VectorParamsAs1DForOutWhenUnconnected=off
  Sel : Outport  Port=2  VectorParamsAs1DForOutWhenUnconnected=off
  wires:
  Valid_in/1 -> Counter_up_to_320/2
  Reset_Count/1 -> Counter_up_to_320/1
  Counter_up_to_320/1 -> Data Type Conversion/1
  Data Type Conversion/1 -> Bit Slice1/1, Bit Slice/1
  Bit Slice1/1 -> Data Type Conversion2/1  "top3Bits"
  Bit Slice/1 -> Data Type Conversion1/1
  Data Type Conversion1/1 -> Addr/1
  Data Type Conversion2/1 -> Sel/1

== system sm_DynamicCompression/dataplane/Avalon Data Processing/Left Channel Processing/recalculate/Nchan_FbankAGC_AID/Addr_Splitter ==
  note: Figure out where 7+ comes from
  note: Addr line contains the local address bits: 0-2^(3+M_bits) -1
  note: Select Line is 000 to 100, if 101 or greater, don't write to any of these blocks
  Register_Addr : Inport
  Bit Slice : hdlsllib/Logic and Bit Operations/Bit Slice  lidx=3+M_bits  ridx=0
      settings: SourceProductName=Simulink  SourceProductBaseCode=SL
  Bit Slice1 : hdlsllib/Logic and Bit Operations/Bit Slice  lidx=6+M_bits  ridx=4+M_bits
      settings: SourceProductName=Simulink  SourceProductBaseCode=SL
  Constant : Constant  Value=5  OutDataTypeStr=fixdt(0,3,0)  SampleTime=-1
  Constant1 : Constant  Value=TABLE_SEL_BYPASS_ENABLE  OutDataTypeStr=boolean  SampleTime=-1
  Data Type Conversion : DataTypeConversion  OutDataTypeStr=fixdt(0,7+M_Bits,0)
  Data Type Conversion1 : DataTypeConversion  OutDataTypeStr=fixdt(0,4+M_bits,0)
  Data Type Conversion2 : DataTypeConversion  OutDataTypeStr=fixdt(0,3,0)
  Switch : Switch  Criteria=u2 ~= 0  Threshold=4
  Addr : Outport  VectorParamsAs1DForOutWhenUnconnected=off
  Sel : Outport  Port=2  VectorParamsAs1DForOutWhenUnconnected=off
  wires:
  Data Type Conversion1/1 -> Addr/1
  Bit Slice1/1 -> Data Type Conversion2/1  "top3Bits"
  Data Type Conversion/1 -> Bit Slice1/1, Bit Slice/1
  Bit Slice/1 -> Data Type Conversion1/1
  Data Type Conversion2/1 -> Switch/1
  Register_Addr/1 -> Data Type Conversion/1
  Switch/1 -> Sel/1
  Constant/1 -> Switch/3
  Constant1/1 -> Switch/2

== system sm_DynamicCompression/dataplane/Avalon Data Processing/Left Channel Processing/recalculate/Nchan_FbankAGC_AID/Compression_1 ==
  note: Delay to account for Comp_Gain_Calc and Compression_Envelope
  note: Make these checks variables?
      | That way its easier to recognize from a
      | matlab workspace
  note: Calculate Compression Gain Needed
  note: Apply to the Envelope
  Sig_Band_1 : Inport
  Table_In : Inport  Port=2
  Table_Sel : Inport  Port=3
  Write_Addr : Inport  Port=4
  Compare To Constant : simulink/Logic and Bit Operations/Compare To Constant  relop===  const=0  OutDataTypeStr=boolean
  Compression_Envelope : Subsystem
  Compression_Gain_Calc : Subsystem
  Constant : Constant  Value=0  OutDataTypeStr=fixdt(1,W_bits,F_bits)  SampleTime=-1
  Data Type Conversion1 : DataTypeConversion  OutDataTypeStr=fixdt(1,W_bits,F_bits)
  Delay : Delay  DelayLength=3
  Product : Product
  Rate Transition : RateTransition  OutPortSampleTime=Ts
  Rate Transition1 : RateTransition  OutPortSampleTime=Ts/FIR_0_Uprate
  Switch : Switch  Criteria=u2 > Threshold  Threshold=4  ZeroCross=off
  Unit Delay : UnitDelay  InitialCondition=1  SampleTime=-1  HasFrameUpgradeWarning=on
  Sig_out : Outport  VectorParamsAs1DForOutWhenUnconnected=off
  wires:
  Compression_Envelope/1(Gain_Out) -> Rate Transition1/1, Unit Delay/1
  Unit Delay/1 -> Compression_Envelope/2(Curr_Gain)
  Product/1 -> Data Type Conversion1/1
  Compare To Constant/1 -> Compression_Gain_Calc/3(Table_Fill_Valid)
  Write_Addr/1 -> Compression_Gain_Calc/2(Write_Addr)
  Table_In/1 -> Compression_Gain_Calc/1(Table_Fill)  "Table_Values"
  Switch/1 -> Delay/1
  Table_Sel/1 -> Compare To Constant/1, Switch/2
  Constant/1 -> Switch/3
  Sig_Band_1/1 -> Compression_Gain_Calc/4(Data_In), Switch/1
  Data Type Conversion1/1 -> Sig_out/1
  Delay/1 -> Product/2
  Compression_Gain_Calc/1(Gain_C_out) -> Rate Transition/1
  Rate Transition/1 -> Compression_Envelope/1(Desired_Gain)
  Rate Transition1/1 -> Product/1

== system sm_DynamicCompression/dataplane/Avalon Data Processing/Left Channel Processing/recalculate/Nchan_FbankAGC_AID/Compression_2 ==
  note: Calculate Compression Gain Needed
  note: Apply to the Envelope
  Sig_Band_1 : Inport
  Table_In : Inport  Port=2
  Table_Sel : Inport  Port=3
  Write_Addr : Inport  Port=4
  Compare To Constant : simulink/Logic and Bit Operations/Compare To Constant  relop===  const=1  OutDataTypeStr=boolean
  Compression_Envelope : Subsystem
  Compression_Gain_Calc : Subsystem
  Constant : Constant  Value=0  OutDataTypeStr=fixdt(1,W_bits,F_bits)  SampleTime=-1
  Data Type Conversion1 : DataTypeConversion  OutDataTypeStr=fixdt(1,W_bits,F_bits)
  Delay : Delay  DelayLength=3
  Product : Product
  Rate Transition1 : RateTransition  OutPortSampleTime=Ts/FIR_0_Uprate
  Rate Transition2 : RateTransition  OutPortSampleTime=Ts
  Switch : Switch  Criteria=u2 > Threshold  Threshold=4  ZeroCross=off
  Unit Delay : UnitDelay  InitialCondition=1  SampleTime=-1  HasFrameUpgradeWarning=on
  Sig_out : Outport  VectorParamsAs1DForOutWhenUnconnected=off
  wires:
  Compression_Envelope/1(Gain_Out) -> Rate Transition1/1, Unit Delay/1
  Unit Delay/1 -> Compression_Envelope/2(Curr_Gain)
  Compare To Constant/1 -> Compression_Gain_Calc/3(Table_Fill_Valid)
  Write_Addr/1 -> Compression_Gain_Calc/2(Write_Addr)
  Table_In/1 -> Compression_Gain_Calc/1(Table_Fill)  "Table_Values"
  Table_Sel/1 -> Compare To Constant/1, Switch/2
  Constant/1 -> Switch/3
  Switch/1 -> Delay/1
  Sig_Band_1/1 -> Compression_Gain_Calc/4(Data_In), Switch/1
  Product/1 -> Data Type Conversion1/1
  Data Type Conversion1/1 -> Sig_out/1
  Delay/1 -> Product/2
  Compression_Gain_Calc/1(Gain_C_out) -> Rate Transition2/1
  Rate Transition1/1 -> Product/1
  Rate Transition2/1 -> Compression_Envelope/1(Desired_Gain)

== system sm_DynamicCompression/dataplane/Avalon Data Processing/Left Channel Processing/recalculate/Nchan_FbankAGC_AID/Compression_3 ==
  note: Calculate Compression Gain Needed
  note: Apply to the Envelope
  Sig_Band_1 : Inport
  Table_In : Inport  Port=2
  Table_Sel : Inport  Port=3
  Write_Addr : Inport  Port=4
  Compare To Constant : simulink/Logic and Bit Operations/Compare To Constant  relop===  const=2  OutDataTypeStr=boolean
  Compression_Envelope : Subsystem
  Compression_Gain_Calc : Subsystem
  Constant : Constant  Value=0  OutDataTypeStr=fixdt(1,W_bits,F_bits)  SampleTime=-1
  Data Type Conversion1 : DataTypeConversion  OutDataTypeStr=fixdt(1,W_bits,F_bits)
  Delay : Delay  DelayLength=3
  Product : Product
  Rate Transition1 : RateTransition  OutPortSampleTime=Ts
  Rate Transition2 : RateTransition  OutPortSampleTime=Ts/FIR_0_Uprate
  Switch : Switch  Criteria=u2 > Threshold  Threshold=4  ZeroCross=off
  Unit Delay : UnitDelay  InitialCondition=1  SampleTime=-1  HasFrameUpgradeWarning=on
  Sig_out : Outport  VectorParamsAs1DForOutWhenUnconnected=off
  wires:
  Compression_Envelope/1(Gain_Out) -> Rate Transition2/1, Unit Delay/1
  Unit Delay/1 -> Compression_Envelope/2(Curr_Gain)
  Compare To Constant/1 -> Compression_Gain_Calc/3(Table_Fill_Valid)
  Write_Addr/1 -> Compression_Gain_Calc/2(Write_Addr)
  Table_In/1 -> Compression_Gain_Calc/1(Table_Fill)  "Table_Values"
  Switch/1 -> Delay/1
  Table_Sel/1 -> Compare To Constant/1, Switch/2
  Constant/1 -> Switch/3
  Sig_Band_1/1 -> Compression_Gain_Calc/4(Data_In), Switch/1
  Product/1 -> Data Type Conversion1/1
  Data Type Conversion1/1 -> Sig_out/1
  Delay/1 -> Product/2
  Compression_Gain_Calc/1(Gain_C_out) -> Rate Transition1/1
  Rate Transition1/1 -> Compression_Envelope/1(Desired_Gain)
  Rate Transition2/1 -> Product/1

== system sm_DynamicCompression/dataplane/Avalon Data Processing/Left Channel Processing/recalculate/Nchan_FbankAGC_AID/Compression_4 ==
  note: Calculate Compression Gain Needed
  note: Apply to the Envelope
  Sig_Band_1 : Inport
  Table_In : Inport  Port=2
  Table_Sel : Inport  Port=3
  Write_Addr : Inport  Port=4
  Compare To Constant : simulink/Logic and Bit Operations/Compare To Constant  relop===  const=3  OutDataTypeStr=boolean
  Compression_Envelope : Subsystem
  Compression_Gain_Calc : Subsystem
  Constant : Constant  Value=0  OutDataTypeStr=fixdt(1,W_bits,F_bits)  SampleTime=-1
  Data Type Conversion1 : DataTypeConversion  OutDataTypeStr=fixdt(1,W_bits,F_bits)
  Delay : Delay  DelayLength=3
  Product : Product
  Rate Transition1 : RateTransition  OutPortSampleTime=Ts
  Rate Transition2 : RateTransition  OutPortSampleTime=Ts/FIR_0_Uprate
  Switch : Switch  Criteria=u2 > Threshold  Threshold=4  ZeroCross=off
  Unit Delay : UnitDelay  InitialCondition=1  SampleTime=-1  HasFrameUpgradeWarning=on
  Sig_out : Outport  VectorParamsAs1DForOutWhenUnconnected=off
  wires:
  Compression_Envelope/1(Gain_Out) -> Rate Transition2/1, Unit Delay/1
  Unit Delay/1 -> Compression_Envelope/2(Curr_Gain)
  Compare To Constant/1 -> Compression_Gain_Calc/3(Table_Fill_Valid)
  Write_Addr/1 -> Compression_Gain_Calc/2(Write_Addr)
  Table_In/1 -> Compression_Gain_Calc/1(Table_Fill)  "Table_Values"
  Switch/1 -> Delay/1
  Table_Sel/1 -> Compare To Constant/1, Switch/2
  Constant/1 -> Switch/3
  Sig_Band_1/1 -> Compression_Gain_Calc/4(Data_In), Switch/1
  Product/1 -> Data Type Conversion1/1
  Data Type Conversion1/1 -> Sig_out/1
  Delay/1 -> Product/2
  Compression_Gain_Calc/1(Gain_C_out) -> Rate Transition1/1
  Rate Transition1/1 -> Compression_Envelope/1(Desired_Gain)
  Rate Transition2/1 -> Product/1

== system sm_DynamicCompression/dataplane/Avalon Data Processing/Left Channel Processing/recalculate/Nchan_FbankAGC_AID/Compression_5 ==
  note: Calculate Compression Gain Needed
  note: Apply to the Envelope
  Sig_Band_1 : Inport
  Table_In : Inport  Port=2
  Table_Sel : Inport  Port=3
  Write_Addr : Inport  Port=4
  Compare To Constant : simulink/Logic and Bit Operations/Compare To Constant  relop===  const=4  OutDataTypeStr=boolean
  Compression_Envelope : Subsystem
  Compression_Gain_Calc : Subsystem
  Constant : Constant  Value=0  OutDataTypeStr=fixdt(1,W_bits,F_bits)  SampleTime=-1
  Data Type Conversion1 : DataTypeConversion  OutDataTypeStr=fixdt(1,W_bits,F_bits)
  Delay : Delay  DelayLength=3
  Product : Product
  Rate Transition1 : RateTransition  OutPortSampleTime=Ts
  Rate Transition2 : RateTransition  OutPortSampleTime=Ts/FIR_0_Uprate
  Switch : Switch  Criteria=u2 > Threshold  Threshold=4  ZeroCross=off
  Unit Delay : UnitDelay  InitialCondition=1  SampleTime=-1  HasFrameUpgradeWarning=on
  Sig_out : Outport  VectorParamsAs1DForOutWhenUnconnected=off
  wires:
  Compression_Envelope/1(Gain_Out) -> Rate Transition2/1, Unit Delay/1
  Unit Delay/1 -> Compression_Envelope/2(Curr_Gain)
  Compare To Constant/1 -> Compression_Gain_Calc/3(Table_Fill_Valid)
  Write_Addr/1 -> Compression_Gain_Calc/2(Write_Addr)
  Table_In/1 -> Compression_Gain_Calc/1(Table_Fill)  "Table_Values"
  Switch/1 -> Delay/1
  Table_Sel/1 -> Compare To Constant/1, Switch/2
  Constant/1 -> Switch/3
  Sig_Band_1/1 -> Compression_Gain_Calc/4(Data_In), Switch/1
  Product/1 -> Data Type Conversion1/1
  Data Type Conversion1/1 -> Sig_out/1
  Delay/1 -> Product/2
  Compression_Gain_Calc/1(Gain_C_out) -> Rate Transition1/1
  Rate Transition1/1 -> Compression_Envelope/1(Desired_Gain)
  Rate Transition2/1 -> Product/1

== system sm_DynamicCompression/dataplane/Avalon Data Processing/Left Channel Processing/recalculate/Nchan_FbankAGC_AID/Static_pFIR ==
  note: consider desired output rate
  note: B_ks will be programmable eventually.
      | For the Conference, they will be preset.
  Data_In : Inport
  Valid_in : Inport  Port=2
  "Addr_Gen " : Subsystem
  Alignment_Delay : UnitDelay  SampleTime=-1  HasFrameUpgradeWarning=on
  Always_read_B2 : Constant  Value=0  OutDataTypeStr=boolean  SampleTime=Ts/FIR_0_Uprate
  B_k_Memory_Block : Subsystem  AncestorBlock=DualPortRam_UNLOCKED/Dual Rate Dual Port RAM1  mask(Dual-rate dual-port RAM){ram_size=FIR_0_Size}
      mask prompts: ram_size "Address port width (2 to 28 bits)"
      mask help: This block simulates a dual-clock dual-port RAM with two data output ports.
      mask init:
      | hdlblkmask_drdpram();
      mask Help: helpview([docroot '/simulink/helptargets.map'],'HDL_dual_rate_dual_port_ram');
  Input_Data_Circular_Buffer : hdlsllib/HDL RAMs/Simple Dual Port RAM  ram_size=FIR_0_Size
      settings: SourceProductName=Simulink  SourceProductBaseCode=SL
  Input_Data_Circular_Buffer_old : Subsystem  Commented=on  AncestorBlock=DualPortRam_UNLOCKED/Dual Rate Dual Port RAM1  mask(Dual-rate dual-port RAM){ram_size=FIR_0_Size}
      mask prompts: ram_size "Address port width (2 to 28 bits)"
      mask help: This block simulates a dual-clock dual-port RAM with two data output ports.
      mask init:
      | hdlblkmask_drdpram();
      mask Help: helpview([docroot '/simulink/helptargets.map'],'HDL_dual_rate_dual_port_ram');
  Multiply_And_Sum : Subsystem
  Never_write_B2 : Constant  Value=0  OutDataTypeStr=fixdt(1,W_bits, F_bits)  SampleTime=Ts/FIR_0_Uprate
  Output_memory : UnitDelay  SampleTime=-1  HasFrameUpgradeWarning=on
  READ_ONLY_1 : Constant  Value=0  OutDataTypeStr=fixdt(1,W_bits, F_bits)  SampleTime=Ts/FIR_0_Uprate
  READ_ONLY_2 : Constant  Value=0  OutDataTypeStr=fixdt(0,FIR_0_Size, 0)  SampleTime=Ts/FIR_0_Uprate
  READ_ONLY_3 : Constant  Value=0  OutDataTypeStr=boolean  SampleTime=Ts/FIR_0_Uprate
  Rate Transition : RateTransition  Commented=on  OutPortSampleTime=Ts
  Reset_Switch : Switch  Criteria=u2 ~= 0
  Terminator7 : Terminator
  Data_out : Outport  VectorParamsAs1DForOutWhenUnconnected=off
  Valid_out : Outport  Port=2  VectorParamsAs1DForOutWhenUnconnected=off
  wires:
  READ_ONLY_2/1 -> B_k_Memory_Block/2(addr_A)
  Always_read_B2/1 -> B_k_Memory_Block/6(we_B)
  B_k_Memory_Block/1(dout_A) -> Terminator7/1
  "Addr_Gen "/3(End_of_sample_calc) -> Alignment_Delay/1
  B_k_Memory_Block/2(dout_B) -> Multiply_And_Sum/3(b_i)  "b_i"
  Reset_Switch/1 -> Output_memory/1
  Multiply_And_Sum/2(Output_Valid) -> Valid_out/1, Reset_Switch/2
  READ_ONLY_1/1 -> B_k_Memory_Block/1(din_A)
  Never_write_B2/1 -> B_k_Memory_Block/4(din_B)
  Input_Data_Circular_Buffer/1 -> Multiply_And_Sum/1(x[n-i])  "x[n-i]"
  "Addr_Gen "/2(Data_History_Rd_addr) -> Input_Data_Circular_Buffer/4
  Valid_in/1 -> Input_Data_Circular_Buffer/3
  Output_memory/1 -> Data_out/1, Reset_Switch/3
  READ_ONLY_3/1 -> B_k_Memory_Block/3(we_A)
  "Addr_Gen "/1(Input_Addr) -> Input_Data_Circular_Buffer/2
  Multiply_And_Sum/1(Filtered_Output) -> Reset_Switch/1
  "Addr_Gen "/4(b_k_addr) -> B_k_Memory_Block/5(addr_B)
  Data_In/1 -> Input_Data_Circular_Buffer/1  "x[n]"
  Alignment_Delay/1 -> Multiply_And_Sum/2(End_of_sample_calc)

== system sm_DynamicCompression/dataplane/Avalon Data Processing/Left Channel Processing/recalculate/Nchan_FbankAGC_AID/Static_pFIR1 ==
  note: B_ks will be programmable eventually.
      | For the Conference, they will be preset.
  note: consider desired output rate
  Data_In : Inport
  Valid_in : Inport  Port=2
  "Addr_Gen " : Subsystem
  Alignment_Delay : UnitDelay  SampleTime=-1  HasFrameUpgradeWarning=on
  Always_read_B2 : Constant  Value=0  OutDataTypeStr=boolean  SampleTime=Ts/FIR_0_Uprate
  B_k_Memory_Block : Subsystem  AncestorBlock=DualPortRam_UNLOCKED/Dual Rate Dual Port RAM1  mask(Dual-rate dual-port RAM){ram_size=FIR_0_Size}
      mask prompts: ram_size "Address port width (2 to 28 bits)"
      mask help: This block simulates a dual-clock dual-port RAM with two data output ports.
      mask init:
      | hdlblkmask_drdpram();
      mask Help: helpview([docroot '/simulink/helptargets.map'],'HDL_dual_rate_dual_port_ram');
  Input_Data_Circular_Buffer : hdlsllib/HDL RAMs/Simple Dual Port RAM  ram_size=FIR_0_Size
      settings: SourceProductName=Simulink  SourceProductBaseCode=SL
  Input_Data_Circular_Buffer_old : Subsystem  Commented=on  AncestorBlock=DualPortRam_UNLOCKED/Dual Rate Dual Port RAM1  mask(Dual-rate dual-port RAM){ram_size=FIR_0_Size}
      mask prompts: ram_size "Address port width (2 to 28 bits)"
      mask help: This block simulates a dual-clock dual-port RAM with two data output ports.
      mask init:
      | hdlblkmask_drdpram();
      mask Help: helpview([docroot '/simulink/helptargets.map'],'HDL_dual_rate_dual_port_ram');
  Multiply_And_Sum : Subsystem
  Never_write_B2 : Constant  Value=0  OutDataTypeStr=fixdt(1,W_bits, F_bits)  SampleTime=Ts/FIR_0_Uprate
  Output_memory : UnitDelay  SampleTime=-1  HasFrameUpgradeWarning=on
  READ_ONLY_1 : Constant  Value=0  OutDataTypeStr=fixdt(1,W_bits, F_bits)  SampleTime=Ts/FIR_0_Uprate
  READ_ONLY_2 : Constant  Value=0  OutDataTypeStr=fixdt(0,FIR_0_Size, 0)  SampleTime=Ts/FIR_0_Uprate
  READ_ONLY_3 : Constant  Value=0  OutDataTypeStr=boolean  SampleTime=Ts/FIR_0_Uprate
  Rate Transition : RateTransition  Commented=on  OutPortSampleTime=Ts
  Reset_Switch : Switch  Criteria=u2 ~= 0
  Terminator7 : Terminator
  Data_out : Outport  VectorParamsAs1DForOutWhenUnconnected=off
  wires:
  Alignment_Delay/1 -> Multiply_And_Sum/2(End_of_sample_calc)
  Data_In/1 -> Input_Data_Circular_Buffer/1  "x[n]"
  "Addr_Gen "/4(b_k_addr) -> B_k_Memory_Block/5(addr_B)
  Multiply_And_Sum/1(Filtered_Output) -> Reset_Switch/1
  "Addr_Gen "/1(Input_Addr) -> Input_Data_Circular_Buffer/2
  READ_ONLY_3/1 -> B_k_Memory_Block/3(we_A)
  Output_memory/1 -> Reset_Switch/3, Data_out/1
  Valid_in/1 -> Input_Data_Circular_Buffer/3
  "Addr_Gen "/2(Data_History_Rd_addr) -> Input_Data_Circular_Buffer/4
  Input_Data_Circular_Buffer/1 -> Multiply_And_Sum/1(x[n-i])  "x[n-i]"
  Never_write_B2/1 -> B_k_Memory_Block/4(din_B)
  READ_ONLY_1/1 -> B_k_Memory_Block/1(din_A)
  Multiply_And_Sum/2(Output_Valid) -> Reset_Switch/2
  Reset_Switch/1 -> Output_memory/1
  B_k_Memory_Block/2(dout_B) -> Multiply_And_Sum/3(b_i)  "b_i"
  "Addr_Gen "/3(End_of_sample_calc) -> Alignment_Delay/1
  B_k_Memory_Block/1(dout_A) -> Terminator7/1
  Always_read_B2/1 -> B_k_Memory_Block/6(we_B)
  READ_ONLY_2/1 -> B_k_Memory_Block/2(addr_A)
